simulink model "Aactuating_lab1"  (R2017b)
settings: Solver=VariableStepAuto  StartTime=0.0  StopTime=10.0  RelTol=1e-3
settings Model: Creator=kamzab95  LastModifiedBy=kamzab95

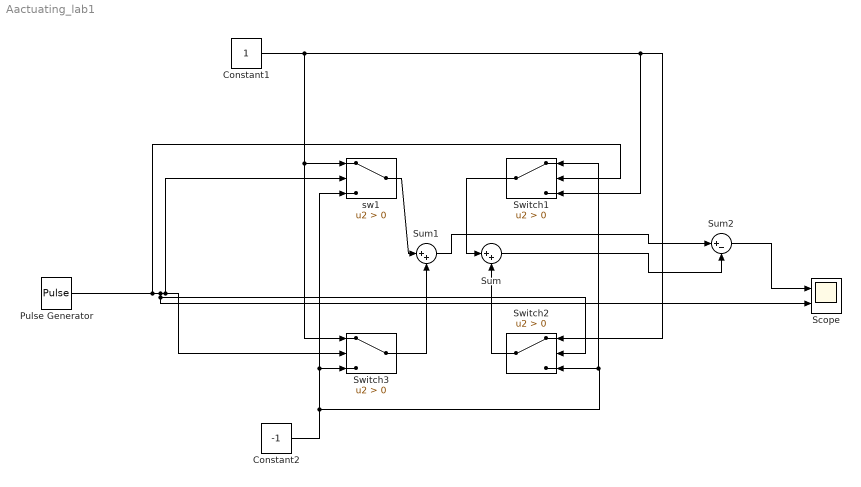
== system Aactuating_lab1 ==
  Constant1 : Constant
  Constant2 : Constant  Value=-1
  Pulse Generator : DiscretePulseGenerator  PulseType=Time based  Period=1  PulseWidth=50
  Scope : Scope  NumInputPorts=2
  Sum : Sum  Inputs=|++
  Sum1 : Sum  Inputs=|++
  Sum2 : Sum  Inputs=|+-
  Switch1 : Switch  Criteria=u2 > Threshold
  Switch2 : Switch  Criteria=u2 > Threshold
  Switch3 : Switch  Criteria=u2 > Threshold
  sw1 : Switch  Criteria=u2 > Threshold
  wires:
  sw1/1 -> Sum1/1
  Switch1/1 -> Sum/1
  Pulse Generator/1 -> Scope/2, Switch2/2, sw1/2, Switch3/2, Switch1/2
  Constant1/1 -> sw1/1, Switch3/1, Switch1/3, Switch2/1
  Sum1/1 -> Sum2/1
  Sum/1 -> Sum2/2
  Sum2/1 -> Scope/1
  Switch3/1 -> Sum1/2
  Switch2/1 -> Sum/2
  Constant2/1 -> Switch1/1, Switch2/3, Switch3/3, sw1/3
